simulink model "sf_if"  (Simulink 6.0)
settings: Solver=ode45  StartTime=0.0  StopTime=10.0  MaxStep=.05  RelTol=1e-3
libraries: simulink x1
settings Model: CovMetricSettings=dcmtr  Creator=The MathWorks Inc.  LastModifiedBy=batserve  ExtModeAutoUpdateStatusClock=off
settings DataIOCC: SignalLoggingName=sigsOut
settings DebuggingCC: CheckExecutionContextPreStartOutputMsg=on  CheckExecutionContextRuntimeOutputMsg=on  SolverPrmCheckMsg=none
settings HardwareCC: TargetUnknown=on

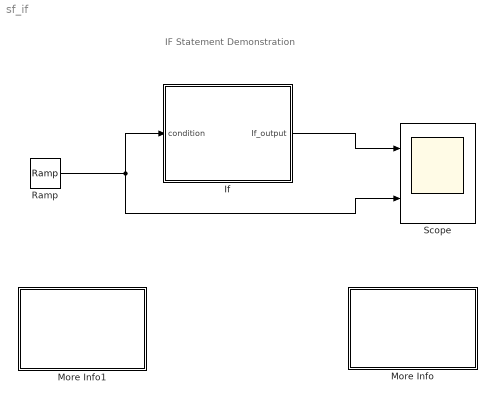
== system sf_if ==
  note: IF Statement Demonstration
  If : Stateflow chart  PropExecContextAcrossSSBoundary=on
  More Info : Subsystem  PropExecContextAcrossSSBoundary=on
      mask Display: disp('Double click\nhere for\ninformation on\nthis demonstration')
  More Info1 : Subsystem  PropExecContextAcrossSSBoundary=on
      settings: OpenFcn=simcad(bdroot);
      mask Display: disp('Double click\nhere for\nSimulink\Stateflow\n Help')
  Ramp : simulink/Sources/Ramp  slope=10  start=0  X0=0
  Scope : Scope  NumInputPorts=2
      settings: TimeRange=10  YMin=-100~0  YMax=400~100
  wires:
  Ramp/1 -> If/1(condition), Scope/2
  If/1(If_output) -> Scope/1

== system sf_if/More Info ==
  note: IF Statement
  note: With the use of flow charts, Stateflow allows you to create C-Code or M-Code statements such as
      | the IF - ELSE statement. This particular demo shows how you can create a simple IF - ELSE
      | statement in Stateflow using an input from Simulink. The equivalent statement in MATLAB is as
      | follows:
      |
      | if condition <= 20
      |     If_output = condition^2;
      | elseif condition > 20 & condition <=50
      |    If_output = 50*sin(condition)
      | else
      |    If_ouptut = condition;
      | end
      |
      | where CONDITION is a ramp input with a slope of  10 simulated for 10 seconds (hence the input
      | vector ranges from 0 to 100 thus covers all of the above conditions).

== system sf_if/More Info1 ==

== stateflow chart If ==
  note: Equivalent M-Code:
      |
      | if condition <= 20
      |     If_output = condition^2;
      | elseif condition > 20 & condition <=50
      |    If_output = 50*sin(condition)
      | else
      |    If_ouptut = condition;
      | end
  (default) -> (junction 4)
  (junction 4) -> (junction 5) : [condition<=20] {If_output=condition^2;}
  (junction 4) -> (junction 5) : {If_output=condition;}
  (junction 4) -> (junction 5) : [condition>20 && condition<=70]
      | {If_output=50*sin(condition);}
  (junction 5) -> (junction 6)
  data: condition input double; If_output output double
